simulink model "constraints_comparison_A_4D_v2_Fc_connected"  (R2017b)
settings: Solver=ode4  StartTime=0.0  StopTime=total_time  FixedStep=0.001  RelTol=1e-3  EnableMultiTasking=on
InitFcn:
  | % clear
  | % clc
  | 
  | wavelet_gen
undefined symbols (not defined in the file or in its folder): acm_aero_model, acm_T_N, breakpoints1, Cm0, Cmde, Cmq, comp_feedback, constraint_type, dail, de, dele, dele_trim, drud, FCdelay, firstimpulsewidth3211, firstimpulsewidthdoublet, Fr_mp_1, Fr_mp_2, Fr_rp_1, Fr_rp_2, ini_acm_de_deg, ini_acm_p_deg_per_s, ini_acm_phi_deg, ini_acm_psi_deg, ini_acm_q_deg_per_s, ini_acm_r_deg_per_s, ini_acm_theta_deg, ini_cmp_de_deg, ini_rig_p_deg_per_s, ini_rig_phi_deg, ini_rig_psi_deg, ini_rig_q_deg_per_s, ini_rig_r_deg_per_s, ini_rig_theta_deg, input_type, K1_svo_acm, K1_svo_cmp, K2_svo_acm, K2_svo_cmp, La, Ma, max_defl_sat_acm, max_defl_sat_cmp, max_rate_sat, max_rate_sat_acm, max_rate_sat_cmp, Na, radius, sigbuilder_block, simstop, theta_trim, thrust_trim, windspeed, Xa, Ya, Za
libraries: aerolibconvert2 x119, simulink x36, sharedtransform x19, vrlib x2
(part 3 of 6)

== system constraints_comparison_A_4D_v2_Fc_connected/Control surface input/5) Dutch roll ==
  note: From the lateral_linear_model.m script:
      | The Dutch roll has a damped natural frequency of 12.9511 rad/s (2.0612 Hz)
      | So the period of the mode is: T = 1/2.0612 = 0.4852 seconds
      |
      | From simulation results:
      | T = 0.4825 seconds
      | f = 2.0725 Hz
  note: Trim (wings level):
      | T = 2.037 N
      | dail = 0 deg
      | dele = -1.22537 deg
      | drud = 0 deg
      | phi = 0 deg
      | theta = 1.612 deg
      | psi = 0 deg
      |
      | Trim (phi = -15 deg):
      | T = 2.225 N
      | dail = -30.39 deg
      | dele = -1.382 deg
      | drud = -36.89 deg
      | phi = -15.01 deg
      | theta = 5.134 deg
      | psi = 11.95 deg
      |
      | Trim (phi = -10 deg):
      | T = 2.026 N
      | dail = -18.93 deg
      | dele = -1.148 deg
      | drud = -22.97 deg
      | phi = -10 deg
      | theta = 2.793 deg
      | psi = 7.106 deg
  note: Trim (wings level)
      | NO THRUST:
      | T = 0 N
      | dail = 0 deg
      | dele = -1.2402 deg
      | drud = 0 deg
      | phi = 0 deg
      | theta = 1.632 deg
      | psi = 0 deg
  Angle Conversion : aerolibconvert2/Angle Conversion  IU=deg  OU=rad
  Angle Conversion1 : aerolibconvert2/Angle Conversion  IU=deg  OU=rad
  Angle Conversion2 : aerolibconvert2/Angle Conversion  IU=deg  OU=rad
  Constant : Constant  Value=0
  Constant2 : Constant  Value=0
  From Workspace : FromWorkspace  VariableName=waveletDR  SampleTime=0  OutputAfterFinalValue=Setting to zero
  Gain : Gain  Commented=on  Gain=0.5
  Gain1 : Gain
  Gain8 : Gain  Gain=3
  Mux : Mux  Inputs=3
  Signal Builder : Subsystem  Tag=STV Subsys  Commented=on  LoadFcn=sigbuilder_block('load');  StartFcn=sigbuilder_block('start');  StopFcn=sigbuilder_block('stop');  ClipboardFcn=sigbuilder_block('clipboard');  mask(Sigbuilder block){tuvar=[0:10]}
      mask help: Simulink:masks:SigbuilderBlock_MD
      mask init:
      | if ~strcmp(get_param(bdroot(gcbh),'SimulationStatus'),'stopped') tuvar = sigbuilder_block('maskInit'); end
      settings: CopyFcn=sigbuilder_block('copy');  DeleteFcn=sigbuilder_block('delete');  ModelCloseFcn=sigbuilder_block('modelClose');  PreSaveFcn=sigbuilder_block('preSave');  PauseFcn=sigbuilder_block('pause');  ContinueFcn=sigbuilder_block('continue');  NameChangeFcn=sigbuilder_block('namechange');  OpenFcn=sigbuilder_block('open',[648.75 96.75 712.5 561.75 ]);  CloseFcn=sigbuilder_block('close');
      mask Display: plot(0, 0, 100, 100,[2, 2, 32, 32, 2], [68, 8, 8, 68, 68],[32, 2], [38, 38], [32, 19, 2],[53, 60, 44], [32, 17, 17, 2],[16, 16, 31, 31]);txt = getActiveGroup(gcbh);text(2, 100, txt,'verticalAlignment', 'top');
  Signal Builder1 : Subsystem  Tag=STV Subsys  LoadFcn=sigbuilder_block('load');  StartFcn=sigbuilder_block('start');  StopFcn=sigbuilder_block('stop');  ClipboardFcn=sigbuilder_block('clipboard');  mask(Sigbuilder block){tuvar=[0:10]}
      mask help: Simulink:masks:SigbuilderBlock_MD
      mask init:
      | if ~strcmp(get_param(bdroot(gcbh),'SimulationStatus'),'stopped') tuvar = sigbuilder_block('maskInit'); end
      settings: CopyFcn=sigbuilder_block('copy');  DeleteFcn=sigbuilder_block('delete');  ModelCloseFcn=sigbuilder_block('modelClose');  PreSaveFcn=sigbuilder_block('preSave');  PauseFcn=sigbuilder_block('pause');  ContinueFcn=sigbuilder_block('continue');  NameChangeFcn=sigbuilder_block('namechange');  OpenFcn=sigbuilder_block('open',[715.5 30.75 718.5 675 ]);  CloseFcn=sigbuilder_block('close');
      mask Display: plot(0, 0, 100, 100,[2, 2, 32, 32, 2], [68, 8, 8, 68, 68],[32, 2], [38, 38], [32, 19, 2],[53, 60, 44], [32, 17, 17, 2],[16, 16, 31, 31]);txt = getActiveGroup(gcbh);text(2, 100, txt,'verticalAlignment', 'top');
  Sum : Sum  Inputs=++|
  Sum1 : Sum  Inputs=++|
  Sum2 : Sum  Inputs=++|
  dail_ini : Constant  Value=0
  dele_ini : Constant  Value=-1.2402
  dele_ini1 : Constant  Value=dele_trim
  drud_ini : Constant  Value=0.000000001
  cs_command (rad) : Outport
  wires:
  Angle Conversion2/1 -> Mux/3  "drud"
  Angle Conversion1/1 -> Mux/2  "dele"
  Angle Conversion/1 -> Mux/1  "dail"
  Mux/1 -> cs_command (rad)/1
  Signal Builder1/1(Signal 1) -> Gain1/1
  Signal Builder/1(Signal 1) -> Gain/1
  Constant/1 -> Sum/2
  Gain8/1 -> Sum2/2
  Constant2/1 -> Sum1/2
  dail_ini/1 -> Sum/1
  dele_ini/1 -> ?
  drud_ini/1 -> Sum2/1
  Sum2/1 -> Angle Conversion2/1
  Sum1/1 -> Angle Conversion1/1
  Sum/1 -> Angle Conversion/1
  dele_ini1/1 -> Sum1/1
  From Workspace/1 -> Gain8/1

== system constraints_comparison_A_4D_v2_Fc_connected/Subsystem14/Aerodynamics lookup ==
  Alpha (deg) : Inport
  1-D Lookup Table : Lookup_n-D  NumberOfTableDimensions=1  BreakpointsForDimension1=breakpoints1  Table=de  DiagnosticForOutOfRangeInput=Warning  InternalRulePriority=Speed  RndMeth=Simplest  InputSameDT=on
  1-D Lookup Table1 : Lookup_n-D  NumberOfTableDimensions=1  BreakpointsForDimension1=breakpoints1  Table=Cm0  DiagnosticForOutOfRangeInput=Warning  InternalRulePriority=Speed  RndMeth=Simplest  InputSameDT=on
  1-D Lookup Table2 : Lookup_n-D  NumberOfTableDimensions=1  BreakpointsForDimension1=breakpoints1  Table=Cmde  DiagnosticForOutOfRangeInput=Warning  InternalRulePriority=Speed  RndMeth=Simplest  InputSameDT=on
  1-D Lookup Table3 : Lookup_n-D  NumberOfTableDimensions=1  BreakpointsForDimension1=breakpoints1  Table=Cmq  DiagnosticForOutOfRangeInput=Warning  InternalRulePriority=Speed  RndMeth=Simplest  InputSameDT=on
  Cm0 : Outport
  Cmde : Outport  Port=2
  de_deg : Outport  Port=3
  Cmq : Outport  Port=4
  wires:
  1-D Lookup Table/1 -> de_deg/1  "de_deg"
  1-D Lookup Table1/1 -> Cm0/1  "Cm0"
  Alpha (deg)/1 -> 1-D Lookup Table3/1, 1-D Lookup Table/1, 1-D Lookup Table2/1, 1-D Lookup Table1/1  "Alpha (deg)"
  1-D Lookup Table3/1 -> Cmq/1  "Cmq"
  1-D Lookup Table2/1 -> Cmde/1  "Cmde"

== system constraints_comparison_A_4D_v2_Fc_connected/Subsystem14/Compensator servo model1 ==
  Command : Inport
  Mot : Gain  Gain=K2_svo_cmp
  Saturation : Saturate  UpperLimit=max_rate_sat_cmp  LowerLimit=-max_rate_sat_cmp
  Sum : Sum  Inputs=|+-
  Sum1 : Sum  Inputs=|+-
  Svo : Gain  Gain=K1_svo_cmp
  kinematic : Subsystem
  Response : Outport
  wires:
  Sum/1 -> Svo/1
  Svo/1 -> Saturation/1
  Sum1/1 -> Mot/1
  Saturation/1 -> Sum1/1
  kinematic/1(de) -> Response/1, Sum/2
  Mot/1 -> kinematic/1(rate_dot)
  kinematic/2(de_dot) -> Sum1/2
  Command/1 -> Sum/1

== system constraints_comparison_A_4D_v2_Fc_connected/Subsystem14/Compensator servo model2 ==
  Command : Inport
  Mot : Gain  Gain=K2_svo_cmp
  Saturation : Saturate  UpperLimit=max_rate_sat_cmp  LowerLimit=-max_rate_sat_cmp
  Sum : Sum  Inputs=|+-
  Sum1 : Sum  Inputs=|+-
  Svo : Gain  Gain=K1_svo_cmp
  kinematic : Subsystem
  Response : Outport
  wires:
  Command/1 -> Sum/1
  kinematic/2(de_dot) -> Sum1/2
  Mot/1 -> kinematic/1(rate_dot)
  kinematic/1(de) -> Sum/2, Response/1
  Saturation/1 -> Sum1/1
  Sum1/1 -> Mot/1
  Svo/1 -> Saturation/1
  Sum/1 -> Svo/1

== system constraints_comparison_A_4D_v2_Fc_connected/Subsystem14/Compensator servo model3 ==
  Command : Inport
  Mot : Gain  Gain=K2_svo_cmp
  Saturation : Saturate  UpperLimit=max_rate_sat_cmp  LowerLimit=-max_rate_sat_cmp
  Sum : Sum  Inputs=|+-
  Sum1 : Sum  Inputs=|+-
  Svo : Gain  Gain=K1_svo_cmp
  kinematic : Subsystem
  Response : Outport
  wires:
  Sum/1 -> Svo/1
  Svo/1 -> Saturation/1
  Sum1/1 -> Mot/1
  Saturation/1 -> Sum1/1
  kinematic/1(de) -> Response/1, Sum/2
  Mot/1 -> kinematic/1(rate_dot)
  kinematic/2(de_dot) -> Sum1/2
  Command/1 -> Sum/1

== system constraints_comparison_A_4D_v2_Fc_connected/Subsystem14/Compensator servo model4 ==
  Command : Inport
  Mot : Gain  Gain=K2_svo_cmp
  Saturation : Saturate  UpperLimit=max_rate_sat_cmp  LowerLimit=-max_rate_sat_cmp
  Sum : Sum  Inputs=|+-
  Sum1 : Sum  Inputs=|+-
  Svo : Gain  Gain=K1_svo_cmp
  kinematic : Subsystem
  Response : Outport
  wires:
  Command/1 -> Sum/1
  kinematic/2(de_dot) -> Sum1/2
  Mot/1 -> kinematic/1(rate_dot)
  kinematic/1(de) -> Sum/2, Response/1
  Saturation/1 -> Sum1/1
  Sum1/1 -> Mot/1
  Svo/1 -> Saturation/1
  Sum/1 -> Svo/1

== system constraints_comparison_A_4D_v2_Fc_connected/Subsystem14/Extracting position vector 1 ==
  In1 : Inport
  MATLAB Function : MATLAB Function  TreatAsAtomicUnit=on
  Out1 : Outport
  wires:
  In1/1 -> MATLAB Function/1(u)
  MATLAB Function/1(y) -> Out1/1

== system constraints_comparison_A_4D_v2_Fc_connected/Subsystem14/Extracting position vector 2 ==
  In1 : Inport
  MATLAB Function : MATLAB Function  TreatAsAtomicUnit=on
  Out1 : Outport
  wires:
  In1/1 -> MATLAB Function/1(u)
  MATLAB Function/1(y) -> Out1/1

== system constraints_comparison_A_4D_v2_Fc_connected/Subsystem14/Extracting position vector 2  ==
  In1 : Inport
  MATLAB Function : MATLAB Function  TreatAsAtomicUnit=on
  Out1 : Outport
  wires:
  MATLAB Function/1(y) -> Out1/1
  In1/1 -> MATLAB Function/1(u)

== system constraints_comparison_A_4D_v2_Fc_connected/Subsystem14/Extracting position vector 3 ==
  In1 : Inport
  MATLAB Function : MATLAB Function  TreatAsAtomicUnit=on
  Out1 : Outport
  wires:
  In1/1 -> MATLAB Function/1(u)
  MATLAB Function/1(y) -> Out1/1

== system constraints_comparison_A_4D_v2_Fc_connected/Subsystem14/Extracting position vector 4 ==
  In1 : Inport
  MATLAB Function : MATLAB Function  TreatAsAtomicUnit=on
  Out1 : Outport
  wires:
  MATLAB Function/1(y) -> Out1/1
  In1/1 -> MATLAB Function/1(u)

== system constraints_comparison_A_4D_v2_Fc_connected/Subsystem14/Extracting position vector 5 ==
  In1 : Inport
  MATLAB Function : MATLAB Function  TreatAsAtomicUnit=on
  Out1 : Outport
  wires:
  MATLAB Function/1(y) -> Out1/1
  In1/1 -> MATLAB Function/1(u)

== system constraints_comparison_A_4D_v2_Fc_connected/Subsystem14/Hawk servo model ==
  note: Above saturation
      | represents voltage
      | saturation
  Command : Inport
  Mot : Gain  Gain=K2_svo_acm
  Saturation : Saturate  UpperLimit=max_rate_sat_acm  LowerLimit=-max_rate_sat_acm
  Sum : Sum  Inputs=|+-
  Sum1 : Sum  Inputs=|+-
  Svo : Gain  Gain=K1_svo_acm
  kinematic : Subsystem
  Response : Outport
  wires:
  Sum/1 -> Svo/1
  Svo/1 -> Saturation/1
  Sum1/1 -> Mot/1
  Saturation/1 -> Sum1/1
  kinematic/1(de) -> Response/1, Sum/2
  Mot/1 -> kinematic/1(rate_dot)
  kinematic/2(de_dot) -> Sum1/2
  Command/1 -> Sum/1

== system constraints_comparison_A_4D_v2_Fc_connected/Subsystem14/Signal Builder ==
  Demux : Demux  Tag=STV Demux  Outputs=1
  FromWs : FromWorkspace  Tag=STV FromWs  VariableName=tuvar  SampleTime=0
      SigBuilderData=|
      | common.afterFinalStr = 'Extrapolate'
      | common.sampleTime = 0
      | dataSet.timeRange = [0 10]
      | dataSet.name = 'Group 1'
      | sbobj.Groups.Name = 'Group 1'
      | sbobj.Groups.Signals.Name = 'Signal 1'
      | sbobj.Groups.Signals.XData = [0 1 1 1.1 1.1 1.2 1.2 10]
      | sbobj.Groups.Signals.YData = [0 0 1 1 -1 -1 0 0]
  Signal 1 : Outport  Tag=STV Outport
  wires:
  Demux/1 -> Signal 1/1
  FromWs/1 -> Demux/1

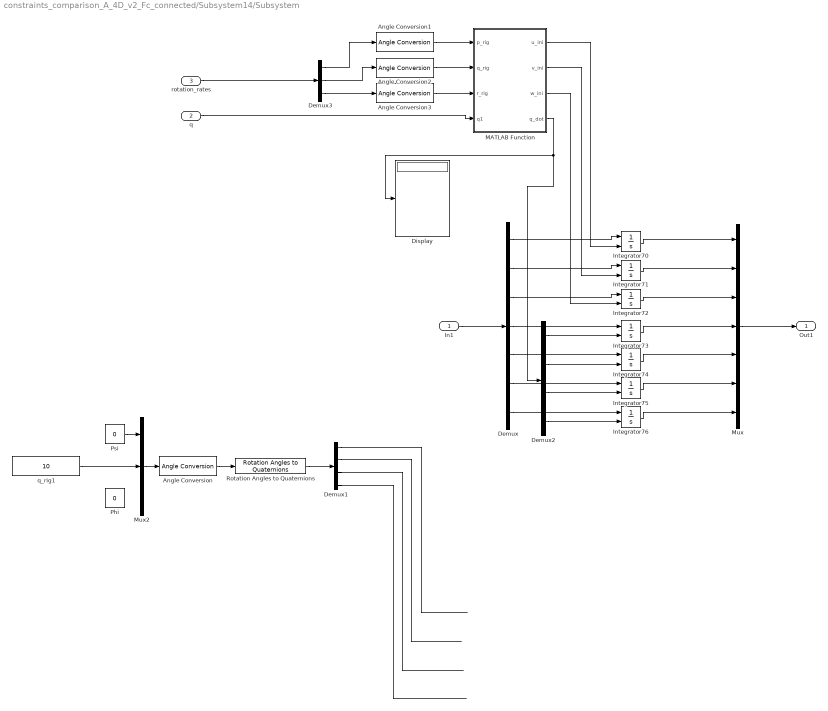
== system constraints_comparison_A_4D_v2_Fc_connected/Subsystem14/Subsystem ==
  In1 : Inport
  q : Inport  Port=2
  rotation_rates : Inport  Port=3
  Angle Conversion{,1..3} (4 alike) : aerolibconvert2/Angle Conversion  IU=deg  OU=rad
  Demux : Demux  Outputs=7
  Demux1 : Demux
  Demux2 : Demux
  Demux3 : Demux  Outputs=3
  Display : Display
  Integrator{70..76} (7 alike) : Integrator  InitialConditionSource=external
  MATLAB Function : MATLAB Function
  Mux : Mux  Inputs=7
  Mux2 : Mux  Inputs=3
  Phi : Constant  Value=0
  Psi : Constant  Value=0
  Rotation Angles to Quaternions : sharedtransform/Rotation Angles to Quaternions  rotationOrder=ZYX
      settings: SourceProductName=Aerospace Blockset  SourceProductBaseCode=AE
  q_rig1 : Constant  Value=10
  Out1 : Outport
  wires:
  Integrator70/1 -> Mux/1
  Integrator71/1 -> Mux/2
  Integrator72/1 -> Mux/3
  Integrator73/1 -> Mux/4
  Integrator74/1 -> Mux/5
  Integrator75/1 -> Mux/6
  Integrator76/1 -> Mux/7
  Demux/1 -> Integrator70/1
  Demux/7 -> Integrator76/1
  Demux/2 -> Integrator71/1
  Demux/3 -> Integrator72/1
  Demux/4 -> Integrator73/1
  Demux/5 -> Integrator74/1
  Demux/6 -> Integrator75/1
  In1/1 -> Demux/1
  Mux/1 -> Out1/1
  MATLAB Function/1(u_ini) -> Integrator70/2
  MATLAB Function/2(v_ini) -> Integrator71/2
  MATLAB Function/3(w_ini) -> Integrator72/2
  rotation_rates/1 -> Demux3/1
  Psi/1 -> Mux2/1
  Mux2/1 -> Angle Conversion/1
  Rotation Angles to Quaternions/1 -> Demux1/1
  Demux1/4 -> ?
  Demux1/1 -> ?
  Demux1/2 -> ?
  Demux1/3 -> ?
  Angle Conversion/1 -> Rotation Angles to Quaternions/1
  Angle Conversion2/1 -> MATLAB Function/2(q_rig)
  q_rig1/1 -> Mux2/2
  q/1 -> MATLAB Function/4(q1)
  Demux2/1 -> Integrator73/2
  Demux2/2 -> Integrator74/2
  Demux2/3 -> Integrator75/2
  Demux2/4 -> Integrator76/2
  MATLAB Function/4(q_dot) -> Demux2/1, Display/1
  Demux3/2 -> Angle Conversion2/1
  Demux3/1 -> Angle Conversion1/1
  Angle Conversion1/1 -> MATLAB Function/1(p_rig)
  Demux3/3 -> Angle Conversion3/1
  Angle Conversion3/1 -> MATLAB Function/3(r_rig)

== system constraints_comparison_A_4D_v2_Fc_connected/Subsystem14/Subsystem1 ==
  In1 : Inport
  rig attitude : Inport  Port=2
  Angle Conversion : aerolibconvert2/Angle Conversion  IU=deg  OU=rad
  Demux : Demux  Outputs=7
  Demux1 : Demux
  Display : Display
  Display1 : Display
  Display2 : Display
  Integrator70 : Integrator  InitialConditionSource=external  InitialCondition=-0.38
  Integrator{71..72,74..76} (5 alike) : Integrator  InitialConditionSource=external
  Integrator73 : Integrator  InitialConditionSource=external  InitialCondition=1
  MATLAB Function : MATLAB Function
  Mux : Mux  Inputs=7
  Quaternions to Rotation Angles : sharedtransform/Quaternions to Rotation Angles  rotationOrder=ZYX
      settings: SourceProductBaseCode=AE
  Rotation Angles to Quaternions : sharedtransform/Rotation Angles to Quaternions  rotationOrder=ZYX
      settings: SourceProductName=Aerospace Blockset  SourceProductBaseCode=AE
  Out1 : Outport
  wires:
  Mux/1 -> Out1/1
  In1/1 -> Demux/1
  Demux/6 -> Integrator75/1
  Demux/5 -> Integrator74/1
  Demux/4 -> Integrator73/1
  Demux/3 -> Integrator72/1
  Demux/2 -> Integrator71/1
  Demux/7 -> Integrator76/1
  Demux/1 -> Integrator70/1
  Integrator76/1 -> Mux/7
  Integrator75/1 -> Mux/6
  Integrator74/1 -> Mux/5
  Integrator73/1 -> Mux/4
  Integrator72/1 -> Mux/3
  Integrator71/1 -> Mux/2
  Integrator70/1 -> Mux/1
  MATLAB Function/1(x_ini) -> Integrator70/2
  MATLAB Function/2(y_ini) -> Integrator71/2
  MATLAB Function/3(z_ini) -> Integrator72/2
  rig attitude/1 -> Angle Conversion/1
  Demux1/4 -> Integrator76/2
  Demux1/1 -> Integrator73/2
  Demux1/2 -> Integrator74/2
  Demux1/3 -> Integrator75/2
  Angle Conversion/1 -> Display1/1, Rotation Angles to Quaternions/1
  Rotation Angles to Quaternions/1 -> Quaternions to Rotation Angles/1, Display/1, MATLAB Function/1(q), Demux1/1
  Quaternions to Rotation Angles/1 -> Display2/1

== system constraints_comparison_A_4D_v2_Fc_connected/Subsystem14/Subsystem10 ==
  In1 : Inport
  q : Inport  Port=2
  rotation_rates : Inport  Port=3
  Angle Conversion1 : aerolibconvert2/Angle Conversion  IU=deg  OU=rad
  Angle Conversion2 : aerolibconvert2/Angle Conversion  IU=deg  OU=rad
  Angle Conversion3 : aerolibconvert2/Angle Conversion  IU=deg  OU=rad
  Demux : Demux  Outputs=7
  Demux1 : Demux
  Demux3 : Demux  Outputs=3
  Display : Display
  Integrator{70..76} (7 alike) : Integrator  InitialConditionSource=external
  MATLAB Function : MATLAB Function
  Mux : Mux  Inputs=7
  Out1 : Outport
  wires:
  Integrator70/1 -> Mux/1
  Integrator71/1 -> Mux/2
  Integrator72/1 -> Mux/3
  Integrator73/1 -> Mux/4
  Integrator74/1 -> Mux/5
  Integrator75/1 -> Mux/6
  Integrator76/1 -> Mux/7
  Demux/1 -> Integrator70/1
  Demux/7 -> Integrator76/1
  Demux/2 -> Integrator71/1
  Demux/3 -> Integrator72/1
  Demux/4 -> Integrator73/1
  Demux/5 -> Integrator74/1
  Demux/6 -> Integrator75/1
  In1/1 -> Demux/1
  Mux/1 -> Out1/1
  MATLAB Function/1(u_ini) -> Integrator70/2
  MATLAB Function/2(v_ini) -> Integrator71/2
  MATLAB Function/3(w_ini) -> Integrator72/2
  rotation_rates/1 -> Demux3/1
  Angle Conversion1/1 -> MATLAB Function/1(p_rig)
  Angle Conversion2/1 -> MATLAB Function/2(q_rig)
  q/1 -> MATLAB Function/4(q1)
  MATLAB Function/4(q_dot) -> Demux1/1, Display/1
  Demux1/4 -> Integrator76/2
  Demux1/3 -> Integrator75/2
  Demux1/2 -> Integrator74/2
  Demux1/1 -> Integrator73/2
  Angle Conversion3/1 -> MATLAB Function/3(r_rig)
  Demux3/3 -> Angle Conversion3/1
  Demux3/2 -> Angle Conversion2/1
  Demux3/1 -> Angle Conversion1/1

== system constraints_comparison_A_4D_v2_Fc_connected/Subsystem14/Subsystem11 ==
  In1 : Inport
  rig attitude : Inport  Port=2
  Angle Conversion : aerolibconvert2/Angle Conversion  IU=deg  OU=rad
  Demux : Demux  Outputs=7
  Demux1 : Demux
  Display : Display
  Integrator70 : Integrator  InitialConditionSource=external  InitialCondition=0.8
  Integrator{71,74..76} (4 alike) : Integrator  InitialConditionSource=external
  Integrator72 : Integrator  InitialConditionSource=external  InitialCondition=0.3183
  Integrator73 : Integrator  InitialConditionSource=external  InitialCondition=1
  MATLAB Function : MATLAB Function
  Mux : Mux  Inputs=7
  Rotation Angles to Quaternions : sharedtransform/Rotation Angles to Quaternions  rotationOrder=ZYX
      settings: SourceProductName=Aerospace Blockset  SourceProductBaseCode=AE
  Terminator : Terminator
  Theta : Constant  Value=0
  Out1 : Outport
  wires:
  Mux/1 -> Out1/1
  In1/1 -> Demux/1
  Demux/6 -> Integrator75/1
  Demux/5 -> Integrator74/1
  Demux/4 -> Integrator73/1
  Demux/3 -> Integrator72/1
  Demux/2 -> Integrator71/1
  Demux/7 -> Integrator76/1
  Demux/1 -> Integrator70/1
  Integrator76/1 -> Mux/7
  Integrator75/1 -> Mux/6
  Integrator74/1 -> Mux/5
  Integrator73/1 -> Mux/4
  Integrator72/1 -> Mux/3
  Integrator71/1 -> Mux/2
  Integrator70/1 -> Mux/1
  Theta/1 -> Terminator/1
  Rotation Angles to Quaternions/1 -> Demux1/1, MATLAB Function/1(q), Display/1
  Demux1/4 -> Integrator76/2
  Demux1/1 -> Integrator73/2
  Demux1/2 -> Integrator74/2
  Demux1/3 -> Integrator75/2
  Angle Conversion/1 -> Rotation Angles to Quaternions/1
  MATLAB Function/1(x_ini) -> Integrator70/2
  MATLAB Function/2(y_ini) -> Integrator71/2
  MATLAB Function/3(z_ini) -> Integrator72/2
  rig attitude/1 -> Angle Conversion/1

== system constraints_comparison_A_4D_v2_Fc_connected/Subsystem14/Subsystem12 ==
  In1 : Inport
  q : Inport  Port=2
  rotation_rates : Inport  Port=3
  Angle Conversion1 : aerolibconvert2/Angle Conversion  IU=deg  OU=rad
  Angle Conversion2 : aerolibconvert2/Angle Conversion  IU=deg  OU=rad
  Angle Conversion3 : aerolibconvert2/Angle Conversion  IU=deg  OU=rad
  Demux : Demux  Outputs=7
  Demux1 : Demux
  Demux3 : Demux  Outputs=3
  Display : Display
  Integrator{70..76} (7 alike) : Integrator  InitialConditionSource=external
  MATLAB Function : MATLAB Function
  Mux : Mux  Inputs=7
  Out1 : Outport
  wires:
  Demux1/1 -> Integrator73/2
  Demux1/2 -> Integrator74/2
  Demux1/3 -> Integrator75/2
  Demux1/4 -> Integrator76/2
  MATLAB Function/4(q_dot) -> Display/1, Demux1/1
  q/1 -> MATLAB Function/4(q1)
  Angle Conversion2/1 -> MATLAB Function/2(q_rig)
  Angle Conversion1/1 -> MATLAB Function/1(p_rig)
  rotation_rates/1 -> Demux3/1
  MATLAB Function/3(w_ini) -> Integrator72/2
  MATLAB Function/2(v_ini) -> Integrator71/2
  MATLAB Function/1(u_ini) -> Integrator70/2
  Mux/1 -> Out1/1
  In1/1 -> Demux/1
  Demux/6 -> Integrator75/1
  Demux/5 -> Integrator74/1
  Demux/4 -> Integrator73/1
  Demux/3 -> Integrator72/1
  Demux/2 -> Integrator71/1
  Demux/7 -> Integrator76/1
  Demux/1 -> Integrator70/1
  Integrator76/1 -> Mux/7
  Integrator75/1 -> Mux/6
  Integrator74/1 -> Mux/5
  Integrator73/1 -> Mux/4
  Integrator72/1 -> Mux/3
  Integrator71/1 -> Mux/2
  Integrator70/1 -> Mux/1
  Angle Conversion3/1 -> MATLAB Function/3(r_rig)
  Demux3/3 -> Angle Conversion3/1
  Demux3/2 -> Angle Conversion2/1
  Demux3/1 -> Angle Conversion1/1

== system constraints_comparison_A_4D_v2_Fc_connected/Subsystem14/Subsystem13 ==
  In1 : Inport
  rig attitude : Inport  Port=2
  Angle Conversion : aerolibconvert2/Angle Conversion  IU=deg  OU=rad
  Demux : Demux  Outputs=7
  Demux1 : Demux
  Display : Display
  Integrator70 : Integrator  InitialConditionSource=external  InitialCondition=0.8
  Integrator{71,74..76} (4 alike) : Integrator  InitialConditionSource=external
  Integrator72 : Integrator  InitialConditionSource=external  InitialCondition=0.1433
  Integrator73 : Integrator  InitialConditionSource=external  InitialCondition=1
  MATLAB Function : MATLAB Function
  Mux : Mux  Inputs=7
  Rotation Angles to Quaternions : sharedtransform/Rotation Angles to Quaternions  rotationOrder=ZYX
      settings: SourceProductName=Aerospace Blockset  SourceProductBaseCode=AE
  Out1 : Outport
  wires:
  Angle Conversion/1 -> Rotation Angles to Quaternions/1
  Demux1/3 -> Integrator75/2
  Demux1/2 -> Integrator74/2
  Demux1/1 -> Integrator73/2
  Demux1/4 -> Integrator76/2
  Integrator70/1 -> Mux/1
  Integrator71/1 -> Mux/2
  Integrator72/1 -> Mux/3
  Integrator73/1 -> Mux/4
  Integrator74/1 -> Mux/5
  Integrator75/1 -> Mux/6
  Integrator76/1 -> Mux/7
  Demux/1 -> Integrator70/1
  Demux/7 -> Integrator76/1
  Demux/2 -> Integrator71/1
  Demux/3 -> Integrator72/1
  Demux/4 -> Integrator73/1
  Demux/5 -> Integrator74/1
  Demux/6 -> Integrator75/1
  In1/1 -> Demux/1
  Mux/1 -> Out1/1
  MATLAB Function/3(z_ini) -> Integrator72/2
  Rotation Angles to Quaternions/1 -> MATLAB Function/1(q), Display/1, Demux1/1
  MATLAB Function/1(x_ini) -> Integrator70/2
  MATLAB Function/2(y_ini) -> Integrator71/2
  rig attitude/1 -> Angle Conversion/1

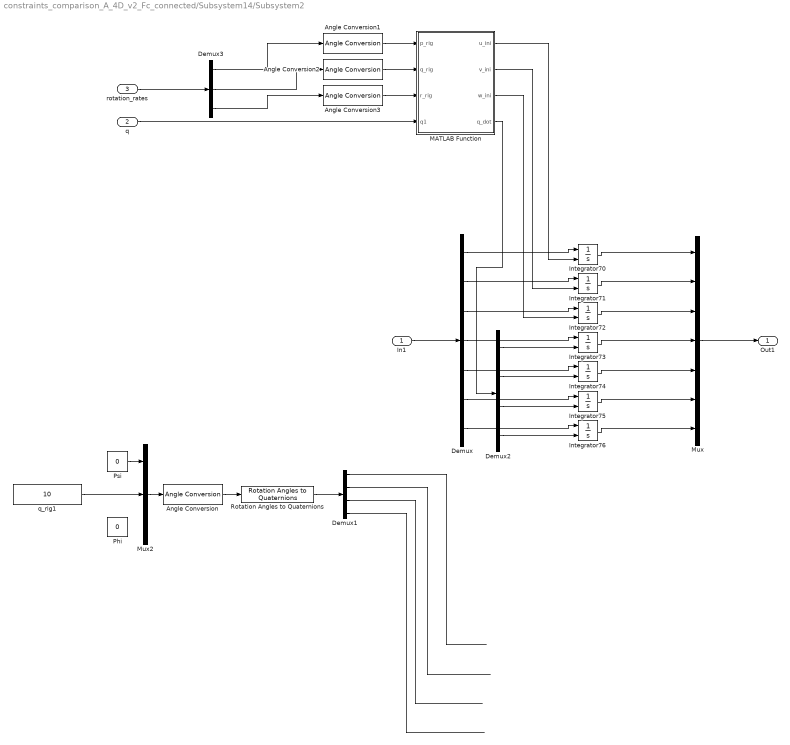
== system constraints_comparison_A_4D_v2_Fc_connected/Subsystem14/Subsystem2 ==
  In1 : Inport
  q : Inport  Port=2
  rotation_rates : Inport  Port=3
  Angle Conversion{,1..3} (4 alike) : aerolibconvert2/Angle Conversion  IU=deg  OU=rad
  Demux : Demux  Outputs=7
  Demux1 : Demux
  Demux2 : Demux
  Demux3 : Demux  Outputs=3
  Integrator{70..76} (7 alike) : Integrator  InitialConditionSource=external
  MATLAB Function : MATLAB Function
  Mux : Mux  Inputs=7
  Mux2 : Mux  Inputs=3
  Phi : Constant  Value=0
  Psi : Constant  Value=0
  Rotation Angles to Quaternions : sharedtransform/Rotation Angles to Quaternions  rotationOrder=ZYX
      settings: SourceProductName=Aerospace Blockset  SourceProductBaseCode=AE
  q_rig1 : Constant  Value=10
  Out1 : Outport
  wires:
  Mux/1 -> Out1/1
  In1/1 -> Demux/1
  Demux/6 -> Integrator75/1
  Demux/5 -> Integrator74/1
  Demux/4 -> Integrator73/1
  Demux/3 -> Integrator72/1
  Demux/2 -> Integrator71/1
  Demux/7 -> Integrator76/1
  Demux/1 -> Integrator70/1
  Integrator76/1 -> Mux/7
  Integrator75/1 -> Mux/6
  Integrator74/1 -> Mux/5
  Integrator73/1 -> Mux/4
  Integrator72/1 -> Mux/3
  Integrator71/1 -> Mux/2
  Integrator70/1 -> Mux/1
  MATLAB Function/1(u_ini) -> Integrator70/2
  MATLAB Function/2(v_ini) -> Integrator71/2
  MATLAB Function/3(w_ini) -> Integrator72/2
  Angle Conversion1/1 -> MATLAB Function/1(p_rig)
  Angle Conversion2/1 -> MATLAB Function/2(q_rig)
  rotation_rates/1 -> Demux3/1
  Psi/1 -> Mux2/1
  Mux2/1 -> Angle Conversion/1
  Rotation Angles to Quaternions/1 -> Demux1/1
  Demux1/4 -> ?
  Demux1/1 -> ?
  Demux1/2 -> ?
  Demux1/3 -> ?
  Angle Conversion/1 -> Rotation Angles to Quaternions/1
  q_rig1/1 -> Mux2/2
  q/1 -> MATLAB Function/4(q1)
  Demux2/1 -> Integrator73/2
  Demux2/2 -> Integrator74/2
  Demux2/3 -> Integrator75/2
  Demux2/4 -> Integrator76/2
  MATLAB Function/4(q_dot) -> Demux2/1
  Demux3/1 -> Angle Conversion1/1
  Demux3/2 -> Angle Conversion2/1
  Angle Conversion3/1 -> MATLAB Function/3(r_rig)
  Demux3/3 -> Angle Conversion3/1

== system constraints_comparison_A_4D_v2_Fc_connected/Subsystem14/Subsystem3 ==
  note: Initial angle of attack -->
  In1 : Inport
  rig attitude : Inport  Port=2
  Angle Conversion : aerolibconvert2/Angle Conversion  IU=deg  OU=rad
  Demux : Demux  Outputs=7
  Demux1 : Demux
  Integrator70 : Integrator  InitialConditionSource=external  InitialCondition=0.2615
  Integrator{71,74..76} (4 alike) : Integrator  InitialConditionSource=external
  Integrator72 : Integrator  InitialConditionSource=external  InitialCondition=0.109
  Integrator73 : Integrator  InitialConditionSource=external  InitialCondition=1
  MATLAB Function : MATLAB Function
  Mux : Mux  Inputs=7
  Rotation Angles to Quaternions : sharedtransform/Rotation Angles to Quaternions  rotationOrder=ZYX
      settings: SourceProductName=Aerospace Blockset  SourceProductBaseCode=AE
  Theta : Constant  Value=0
  Out1 : Outport
  wires:
  Integrator70/1 -> Mux/1
  Integrator71/1 -> Mux/2
  Integrator72/1 -> Mux/3
  Integrator73/1 -> Mux/4
  Integrator74/1 -> Mux/5
  Integrator75/1 -> Mux/6
  Integrator76/1 -> Mux/7
  Demux/1 -> Integrator70/1
  Demux/7 -> Integrator76/1
  Demux/2 -> Integrator71/1
  Demux/3 -> Integrator72/1
  Demux/4 -> Integrator73/1
  Demux/5 -> Integrator74/1
  Demux/6 -> Integrator75/1
  In1/1 -> Demux/1
  Mux/1 -> Out1/1
  MATLAB Function/1(x_ini) -> Integrator70/2
  MATLAB Function/2(y_ini) -> Integrator71/2
  MATLAB Function/3(z_ini) -> Integrator72/2
  Demux1/4 -> Integrator76/2
  Demux1/1 -> Integrator73/2
  Demux1/2 -> Integrator74/2
  Demux1/3 -> Integrator75/2
  Angle Conversion/1 -> Rotation Angles to Quaternions/1
  Rotation Angles to Quaternions/1 -> MATLAB Function/1(q), Demux1/1
  rig attitude/1 -> Angle Conversion/1

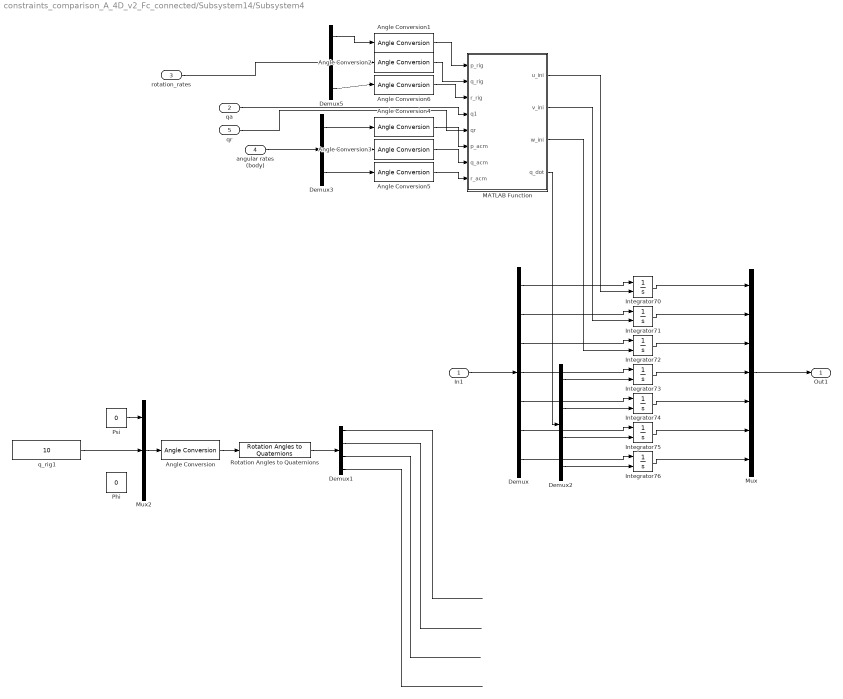
== system constraints_comparison_A_4D_v2_Fc_connected/Subsystem14/Subsystem4 ==
  In1 : Inport
  qa : Inport  Port=2
  rotation_rates : Inport  Port=3
  angular rates (body) : Inport  Port=4
  qr : Inport  Port=5
  Angle Conversion{,1..6} (7 alike) : aerolibconvert2/Angle Conversion  IU=deg  OU=rad
  Demux : Demux  Outputs=7
  Demux1 : Demux
  Demux2 : Demux
  Demux3 : Demux  Outputs=3
  Demux5 : Demux  Outputs=3
  Integrator{70..76} (7 alike) : Integrator  InitialConditionSource=external
  MATLAB Function : MATLAB Function
  Mux : Mux  Inputs=7
  Mux2 : Mux  Inputs=3
  Phi : Constant  Value=0
  Psi : Constant  Value=0
  Rotation Angles to Quaternions : sharedtransform/Rotation Angles to Quaternions  rotationOrder=ZYX
      settings: SourceProductName=Aerospace Blockset  SourceProductBaseCode=AE
  q_rig1 : Constant  Value=10
  Out1 : Outport
  wires:
  Integrator70/1 -> Mux/1
  Integrator71/1 -> Mux/2
  Integrator72/1 -> Mux/3
  Integrator73/1 -> Mux/4
  Integrator74/1 -> Mux/5
  Integrator75/1 -> Mux/6
  Integrator76/1 -> Mux/7
  Demux/1 -> Integrator70/1
  Demux/7 -> Integrator76/1
  Demux/2 -> Integrator71/1
  Demux/3 -> Integrator72/1
  Demux/4 -> Integrator73/1
  Demux/5 -> Integrator74/1
  Demux/6 -> Integrator75/1
  In1/1 -> Demux/1
  Mux/1 -> Out1/1
  MATLAB Function/1(u_ini) -> Integrator70/2
  MATLAB Function/2(v_ini) -> Integrator71/2
  MATLAB Function/3(w_ini) -> Integrator72/2
  Angle Conversion1/1 -> MATLAB Function/1(p_rig)
  Angle Conversion2/1 -> MATLAB Function/2(q_rig)
  rotation_rates/1 -> Demux5/1
  Psi/1 -> Mux2/1
  Mux2/1 -> Angle Conversion/1
  Rotation Angles to Quaternions/1 -> Demux1/1
  Demux1/4 -> ?
  Demux1/1 -> ?
  Demux1/2 -> ?
  Demux1/3 -> ?
  Angle Conversion/1 -> Rotation Angles to Quaternions/1
  q_rig1/1 -> Mux2/2
  qa/1 -> MATLAB Function/4(q1)
  Demux2/1 -> Integrator73/2
  Demux2/2 -> Integrator74/2
  Demux2/3 -> Integrator75/2
  Demux2/4 -> Integrator76/2
  MATLAB Function/4(q_dot) -> Demux2/1
  Angle Conversion3/1 -> MATLAB Function/7(q_acm)
  angular rates (body)/1 -> Demux3/1
  Angle Conversion4/1 -> MATLAB Function/6(p_acm)
  Angle Conversion5/1 -> MATLAB Function/8(r_acm)
  Demux3/3 -> Angle Conversion5/1
  Demux3/1 -> Angle Conversion4/1
  Demux3/2 -> Angle Conversion3/1
  Angle Conversion6/1 -> MATLAB Function/3(r_rig)
  Demux5/1 -> Angle Conversion1/1
  Demux5/2 -> Angle Conversion2/1
  Demux5/3 -> Angle Conversion6/1
  qr/1 -> MATLAB Function/5(qr)

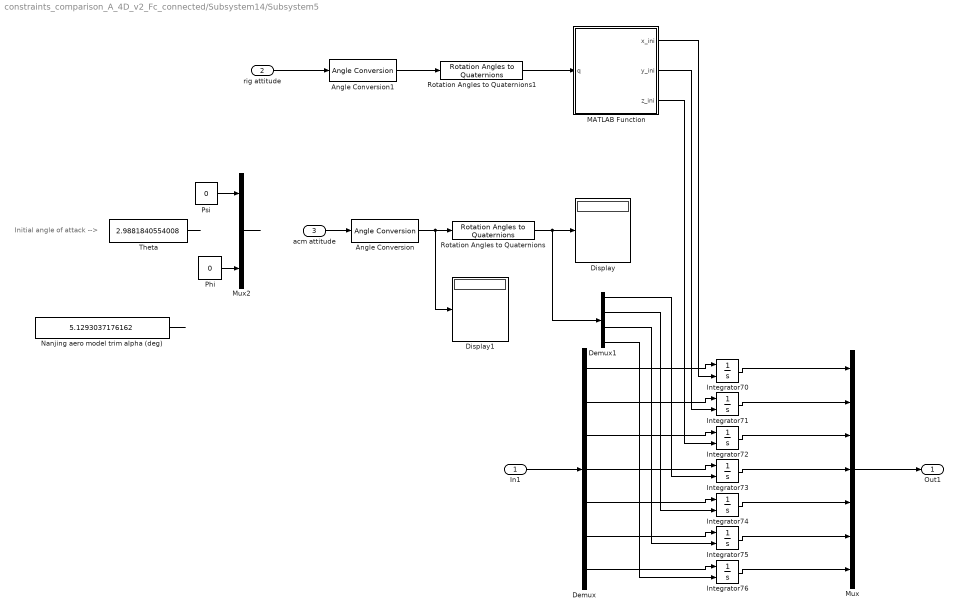
== system constraints_comparison_A_4D_v2_Fc_connected/Subsystem14/Subsystem5 ==
  note: Initial angle of attack -->
  In1 : Inport
  rig attitude : Inport  Port=2
  acm attitude : Inport  Port=3
  Angle Conversion : aerolibconvert2/Angle Conversion  IU=deg  OU=rad
  Angle Conversion1 : aerolibconvert2/Angle Conversion  IU=deg  OU=rad
  Demux : Demux  Outputs=7
  Demux1 : Demux
  Display : Display
  Display1 : Display
  Integrator70 : Integrator  InitialConditionSource=external  InitialCondition=0.8
  Integrator{71..72,74..76} (5 alike) : Integrator  InitialConditionSource=external
  Integrator73 : Integrator  InitialConditionSource=external  InitialCondition=1
  MATLAB Function : MATLAB Function
  Mux : Mux  Inputs=7
  Mux2 : Mux  Inputs=3
  Nanjing aero model trim alpha (deg) : Constant  Value=5.1293037176162
  Phi : Constant  Value=0
  Psi : Constant  Value=0
  Rotation Angles to Quaternions : sharedtransform/Rotation Angles to Quaternions  rotationOrder=ZYX
      settings: SourceProductName=Aerospace Blockset  SourceProductBaseCode=AE
  Rotation Angles to Quaternions1 : sharedtransform/Rotation Angles to Quaternions  rotationOrder=ZYX
      settings: SourceProductName=Aerospace Blockset  SourceProductBaseCode=AE
  Theta : Constant  Value=2.9881840554008
  Out1 : Outport
  wires:
  Mux/1 -> Out1/1
  In1/1 -> Demux/1
  Demux/6 -> Integrator75/1
  Demux/5 -> Integrator74/1
  Demux/4 -> Integrator73/1
  Demux/3 -> Integrator72/1
  Demux/2 -> Integrator71/1
  Demux/7 -> Integrator76/1
  Demux/1 -> Integrator70/1
  Integrator76/1 -> Mux/7
  Integrator75/1 -> Mux/6
  Integrator74/1 -> Mux/5
  Integrator73/1 -> Mux/4
  Integrator72/1 -> Mux/3
  Integrator71/1 -> Mux/2
  Integrator70/1 -> Mux/1
  Phi/1 -> Mux2/3
  Psi/1 -> Mux2/1
  Mux2/1 -> ?
  Rotation Angles to Quaternions/1 -> Demux1/1, Display/1
  Demux1/4 -> Integrator76/2
  Demux1/1 -> Integrator73/2
  Demux1/2 -> Integrator74/2
  Demux1/3 -> Integrator75/2
  Angle Conversion/1 -> Display1/1, Rotation Angles to Quaternions/1
  Nanjing aero model trim alpha (deg)/1 -> ?
  MATLAB Function/1(x_ini) -> Integrator70/2
  MATLAB Function/2(y_ini) -> Integrator71/2
  MATLAB Function/3(z_ini) -> Integrator72/2
  Theta/1 -> ?
  Angle Conversion1/1 -> Rotation Angles to Quaternions1/1
  rig attitude/1 -> Angle Conversion1/1
  acm attitude/1 -> Angle Conversion/1
  Rotation Angles to Quaternions1/1 -> MATLAB Function/1(q)

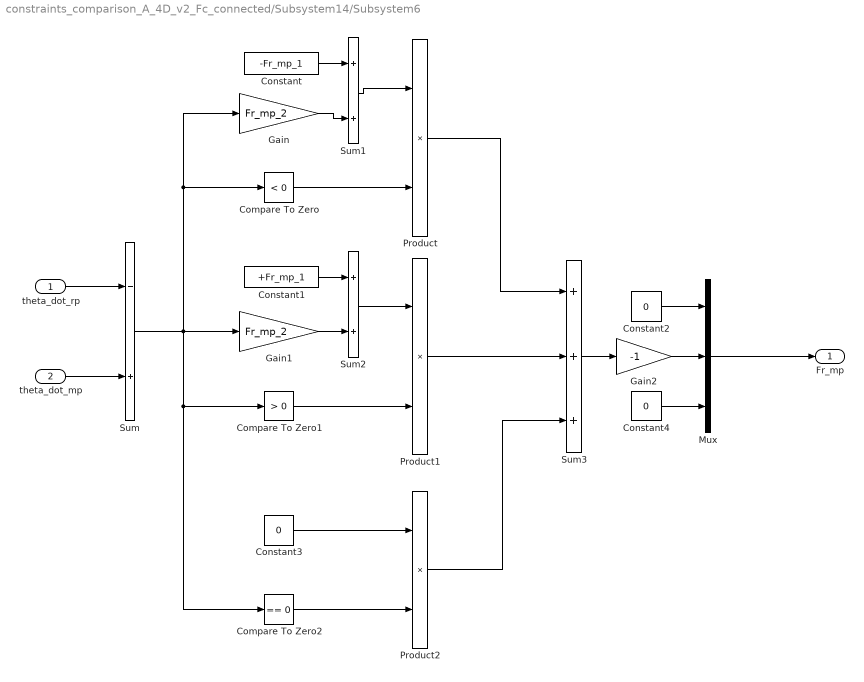
== system constraints_comparison_A_4D_v2_Fc_connected/Subsystem14/Subsystem6 ==
  theta_dot_rp : Inport
  theta_dot_mp : Inport  Port=2
  Compare To Zero : simulink/Logic and Bit Operations/Compare To Zero  relop=<  OutDataTypeStr=boolean
  Compare To Zero1 : simulink/Logic and Bit Operations/Compare To Zero  relop=>  OutDataTypeStr=boolean
  Compare To Zero2 : simulink/Logic and Bit Operations/Compare To Zero  relop===  OutDataTypeStr=boolean
  Constant : Constant  Value=-Fr_mp_1
  Constant1 : Constant  Value=+Fr_mp_1
  Constant2 : Constant  Value=0
  Constant3 : Constant  Value=0
  Constant4 : Constant  Value=0
  Gain : Gain  Gain=Fr_mp_2
  Gain1 : Gain  Gain=Fr_mp_2
  Gain2 : Gain  Gain=-1
  Mux : Mux  Inputs=3
  Product : Product
  Product1 : Product
  Product2 : Product
  Sum : Sum  Inputs=-+
  Sum1 : Sum
  Sum2 : Sum
  Sum3 : Sum  Inputs=+++
  Fr_mp : Outport
  wires:
  theta_dot_rp/1 -> Sum/1
  theta_dot_mp/1 -> Sum/2
  Compare To Zero/1 -> Product/2
  Compare To Zero1/1 -> Product1/2
  Constant/1 -> Sum1/1
  Gain/1 -> Sum1/2
  Sum/1 -> Gain/1, Compare To Zero/1, Compare To Zero2/1, Compare To Zero1/1, Gain1/1
  Sum1/1 -> Product/1
  Constant1/1 -> Sum2/1
  Gain1/1 -> Sum2/2
  Sum2/1 -> Product1/1
  Compare To Zero2/1 -> Product2/2
  Constant4/1 -> Mux/3
  Constant2/1 -> Mux/1
  Mux/1 -> Fr_mp/1
  Constant3/1 -> Product2/1
  Product/1 -> Sum3/1
  Product1/1 -> Sum3/2
  Product2/1 -> Sum3/3
  Sum3/1 -> Gain2/1
  Gain2/1 -> Mux/2

== system constraints_comparison_A_4D_v2_Fc_connected/Subsystem14/Subsystem7 ==
  theta_dot_rp : Inport
  Compare To Zero : simulink/Logic and Bit Operations/Compare To Zero  relop=<  OutDataTypeStr=boolean
  Compare To Zero1 : simulink/Logic and Bit Operations/Compare To Zero  relop=>  OutDataTypeStr=boolean
  Compare To Zero2 : simulink/Logic and Bit Operations/Compare To Zero  relop===  OutDataTypeStr=boolean
  Constant : Constant  Value=-Fr_rp_1
  Constant1 : Constant  Value=+Fr_rp_1
  Constant2 : Constant  Value=0
  Constant3 : Constant  Value=0
  Constant4 : Constant  Value=0
  Gain : Gain  Gain=Fr_rp_2
  Gain1 : Gain  Gain=Fr_rp_2
  Gain2 : Gain  Gain=-1
  Mux : Mux  Inputs=3
  Product : Product
  Product1 : Product
  Product2 : Product
  Sum1 : Sum
  Sum2 : Sum
  Sum3 : Sum  Inputs=+++
  Fr_mp : Outport
  wires:
  Gain2/1 -> Mux/2
  Sum3/1 -> Gain2/1
  Product2/1 -> Sum3/3
  Product1/1 -> Sum3/2
  Product/1 -> Sum3/1
  Constant3/1 -> Product2/1
  Mux/1 -> Fr_mp/1
  Constant2/1 -> Mux/1
  Constant4/1 -> Mux/3
  Compare To Zero2/1 -> Product2/2
  Sum2/1 -> Product1/1
  Gain1/1 -> Sum2/2
  Constant1/1 -> Sum2/1
  Sum1/1 -> Product/1
  theta_dot_rp/1 -> Gain1/1, Compare To Zero1/1, Compare To Zero2/1, Compare To Zero/1, Gain/1
  Gain/1 -> Sum1/2
  Constant/1 -> Sum1/1
  Compare To Zero1/1 -> Product1/2
  Compare To Zero/1 -> Product/2

== system constraints_comparison_A_4D_v2_Fc_connected/Subsystem14/Subsystem8 ==
  In1 : Inport
  Demux : Demux  Outputs=7
  Integrator{70..76} (7 alike) : Integrator
  Mux : Mux  Inputs=7
  Out1 : Outport
  wires:
  Mux/1 -> Out1/1
  In1/1 -> Demux/1
  Demux/6 -> Integrator75/1
  Demux/5 -> Integrator74/1
  Demux/4 -> Integrator73/1
  Demux/3 -> Integrator72/1
  Demux/2 -> Integrator71/1
  Demux/7 -> Integrator76/1
  Demux/1 -> Integrator70/1
  Integrator76/1 -> Mux/7
  Integrator75/1 -> Mux/6
  Integrator74/1 -> Mux/5
  Integrator73/1 -> Mux/4
  Integrator72/1 -> Mux/3
  Integrator71/1 -> Mux/2
  Integrator70/1 -> Mux/1

== system constraints_comparison_A_4D_v2_Fc_connected/Subsystem14/Subsystem9 ==
  In1 : Inport
  Angle Conversion : aerolibconvert2/Angle Conversion  IU=deg  OU=rad
  Demux : Demux  Outputs=7
  Demux1 : Demux
  Display : Display
  Integrator70 : Integrator  InitialCondition=-0.672
  Integrator71 : Integrator
  Integrator72 : Integrator
  Integrator73 : Integrator  InitialConditionSource=external  InitialCondition=1
  Integrator74 : Integrator  InitialConditionSource=external
  Integrator75 : Integrator  InitialConditionSource=external
  Integrator76 : Integrator  InitialConditionSource=external
  Mux : Mux  Inputs=7
  Mux2 : Mux  Inputs=3
  Phi : Constant  Value=0
  Psi : Constant  Value=0
  Rotation Angles to Quaternions : sharedtransform/Rotation Angles to Quaternions  rotationOrder=ZYX
      settings: SourceProductName=Aerospace Blockset  SourceProductBaseCode=AE
  Theta : Constant  Value=0
  Out1 : Outport
  wires:
  Angle Conversion/1 -> Rotation Angles to Quaternions/1
  Demux1/3 -> Integrator75/2
  Demux1/2 -> Integrator74/2
  Demux1/1 -> Integrator73/2
  Demux1/4 -> Integrator76/2
  Rotation Angles to Quaternions/1 -> Display/1, Demux1/1
  Mux2/1 -> Angle Conversion/1
  Phi/1 -> Mux2/1
  Psi/1 -> Mux2/3
  Theta/1 -> Mux2/2
  Integrator70/1 -> Mux/1
  Integrator71/1 -> Mux/2
  Integrator72/1 -> Mux/3
  Integrator73/1 -> Mux/4
  Integrator74/1 -> Mux/5
  Integrator75/1 -> Mux/6
  Integrator76/1 -> Mux/7
  Demux/1 -> Integrator70/1
  Demux/7 -> Integrator76/1
  Demux/2 -> Integrator71/1
  Demux/3 -> Integrator72/1
  Demux/4 -> Integrator73/1
  Demux/5 -> Integrator74/1
  Demux/6 -> Integrator75/1
  In1/1 -> Demux/1
  Mux/1 -> Out1/1

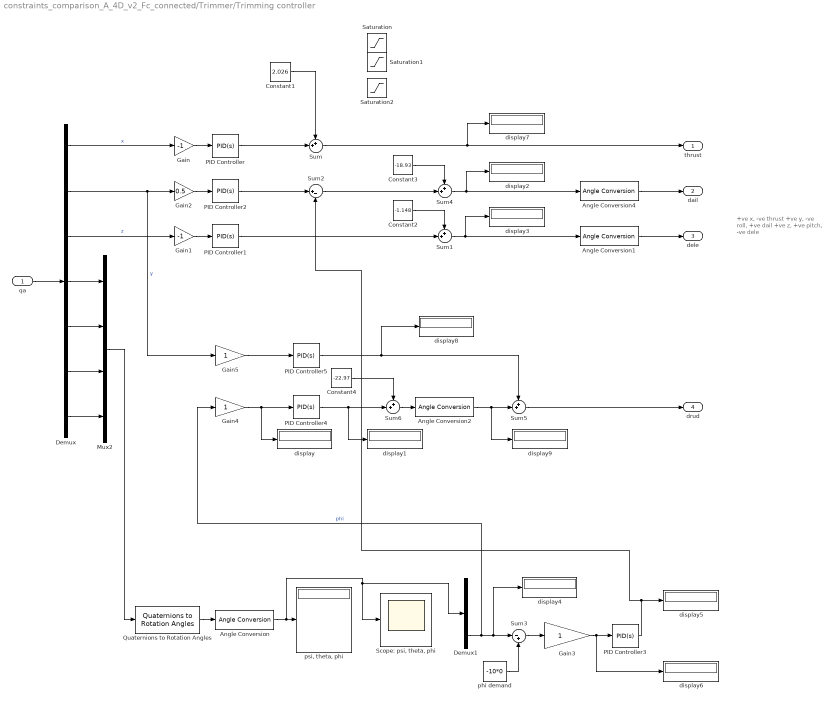
== system constraints_comparison_A_4D_v2_Fc_connected/Trimmer/Trimming controller ==
  note: +ve x, -ve thrust
      |
      | +ve y, -ve roll, +ve dail
      |
      | +ve z, +ve pitch, -ve dele
  qa : Inport
  Angle Conversion : aerolibconvert2/Angle Conversion  IU=rad  OU=deg
  Angle Conversion1 : aerolibconvert2/Angle Conversion  IU=deg  OU=rad
  Angle Conversion2 : aerolibconvert2/Angle Conversion  IU=deg  OU=rad
  Angle Conversion4 : aerolibconvert2/Angle Conversion  IU=deg  OU=rad
  Constant1 : Constant  Value=2.026
  Constant2 : Constant  Value=-1.148
  Constant3 : Constant  Value=-18.93
  Constant4 : Constant  Value=-22.97
  Demux : Demux  Outputs=7
  Demux1 : Demux  Outputs=3
  Gain : Gain  Gain=-1
  Gain1 : Gain  Gain=-1
  Gain2 : Gain  Gain=0.5
  Gain3 : Gain
  Gain4 : Gain
  Gain5 : Gain
  Mux2 : Mux
  PID Controller : simulink/Continuous/PID Controller  Controller=PID  TimeDomain=Continuous-time  SampleTime=-1  IntegratorMethod=Forward Euler  FilterMethod=Forward Euler  Form=Parallel  UseFilter=on  ControllerParametersSource=internal  P=2  I=0.5  D=1  N=100  InitialConditionSource=internal  InitialConditionForIntegrator=0  InitialConditionForFilter=0  ExternalReset=none  LimitOutput=off  UpperSaturationLimit=inf  LowerSaturationLimit=-inf  LinearizeAsGain=on  AntiWindupMode=none  Kb=1  TrackingMode=off  Kt=1  PParamMin=[]  PParamMax=[]  IParamMin=[]  IParamMax=[]  DParamMin=[]  DParamMax=[]  NParamMin=[]  NParamMax=[]  KbParamMin=[]  KbParamMax=[]  KtParamMin=[]  KtParamMax=[]  POutMin=[]  POutMax=[]  IOutMin=[]  IOutMax=[]  DOutMin=[]  DOutMax=[]  NOutMin=[]  NOutMax=[]  KbOutMin=[]  KbOutMax=[]  KtOutMin=[]  KtOutMax=[]  IntegratorOutMin=[]  IntegratorOutMax=[]  FilterOutMin=[]  FilterOutMax=[]  SumOutMin=[]  SumOutMax=[]  SumI1OutMin=[]  SumI1OutMax=[]  SumI2OutMin=[]  SumI2OutMax=[]  SumI3OutMin=[]  SumI3OutMax=[]  SumDOutMin=[]  SumDOutMax=[]  SaturationOutMin=[]  SaturationOutMax=[]  IntegratorContinuousStateAttributes=''  IntegratorStateMustResolveToSignalObject=off  IntegratorRTWStateStorageClass=Auto  FilterContinuousStateAttributes=''  FilterStateMustResolveToSignalObject=off  FilterRTWStateStorageClass=Auto  DifferentiatorICPrevScaledInput=0  DifferentiatorOutMin=[]  DifferentiatorOutMax=[]  InitialConditionSetting=State (most efficient)  FilterDiffOutCoefMin=[]  FilterDiffOutCoefMax=[]  SumDenOutMin=[]  SumDenOutMax=[]  SumNumOutMin=[]  SumNumOutMax=[]  ReciprocalOutMin=[]  ReciprocalOutMax=[]  DivideOutMin=[]  DivideOutMax=[]  TunerSelectOption=Transfer Function Based (PID Tuner App)
  PID Controller1 : simulink/Continuous/PID Controller  Controller=PID  TimeDomain=Continuous-time  SampleTime=-1  IntegratorMethod=Forward Euler  FilterMethod=Forward Euler  Form=Parallel  UseFilter=on  ControllerParametersSource=internal  P=2  I=0.5  D=1  N=100  InitialConditionSource=internal  InitialConditionForIntegrator=0  InitialConditionForFilter=0  ExternalReset=none  LimitOutput=off  UpperSaturationLimit=inf  LowerSaturationLimit=-inf  LinearizeAsGain=on  AntiWindupMode=none  Kb=1  TrackingMode=off  Kt=1  PParamMin=[]  PParamMax=[]  IParamMin=[]  IParamMax=[]  DParamMin=[]  DParamMax=[]  NParamMin=[]  NParamMax=[]  KbParamMin=[]  KbParamMax=[]  KtParamMin=[]  KtParamMax=[]  POutMin=[]  POutMax=[]  IOutMin=[]  IOutMax=[]  DOutMin=[]  DOutMax=[]  NOutMin=[]  NOutMax=[]  KbOutMin=[]  KbOutMax=[]  KtOutMin=[]  KtOutMax=[]  IntegratorOutMin=[]  IntegratorOutMax=[]  FilterOutMin=[]  FilterOutMax=[]  SumOutMin=[]  SumOutMax=[]  SumI1OutMin=[]  SumI1OutMax=[]  SumI2OutMin=[]  SumI2OutMax=[]  SumI3OutMin=[]  SumI3OutMax=[]  SumDOutMin=[]  SumDOutMax=[]  SaturationOutMin=[]  SaturationOutMax=[]  IntegratorContinuousStateAttributes=''  IntegratorStateMustResolveToSignalObject=off  IntegratorRTWStateStorageClass=Auto  FilterContinuousStateAttributes=''  FilterStateMustResolveToSignalObject=off  FilterRTWStateStorageClass=Auto  DifferentiatorICPrevScaledInput=0  DifferentiatorOutMin=[]  DifferentiatorOutMax=[]  InitialConditionSetting=State (most efficient)  FilterDiffOutCoefMin=[]  FilterDiffOutCoefMax=[]  SumDenOutMin=[]  SumDenOutMax=[]  SumNumOutMin=[]  SumNumOutMax=[]  ReciprocalOutMin=[]  ReciprocalOutMax=[]  DivideOutMin=[]  DivideOutMax=[]  TunerSelectOption=Transfer Function Based (PID Tuner App)
  PID Controller2 : simulink/Continuous/PID Controller  Controller=PID  TimeDomain=Continuous-time  SampleTime=-1  IntegratorMethod=Forward Euler  FilterMethod=Forward Euler  Form=Parallel  UseFilter=on  ControllerParametersSource=internal  P=0.1  I=0.1  D=0.5  N=100  InitialConditionSource=internal  InitialConditionForIntegrator=0  InitialConditionForFilter=0  ExternalReset=none  LimitOutput=off  UpperSaturationLimit=inf  LowerSaturationLimit=-inf  LinearizeAsGain=on  AntiWindupMode=none  Kb=1  TrackingMode=off  Kt=1  PParamMin=[]  PParamMax=[]  IParamMin=[]  IParamMax=[]  DParamMin=[]  DParamMax=[]  NParamMin=[]  NParamMax=[]  KbParamMin=[]  KbParamMax=[]  KtParamMin=[]  KtParamMax=[]  POutMin=[]  POutMax=[]  IOutMin=[]  IOutMax=[]  DOutMin=[]  DOutMax=[]  NOutMin=[]  NOutMax=[]  KbOutMin=[]  KbOutMax=[]  KtOutMin=[]  KtOutMax=[]  IntegratorOutMin=[]  IntegratorOutMax=[]  FilterOutMin=[]  FilterOutMax=[]  SumOutMin=[]  SumOutMax=[]  SumI1OutMin=[]  SumI1OutMax=[]  SumI2OutMin=[]  SumI2OutMax=[]  SumI3OutMin=[]  SumI3OutMax=[]  SumDOutMin=[]  SumDOutMax=[]  SaturationOutMin=[]  SaturationOutMax=[]  IntegratorContinuousStateAttributes=''  IntegratorStateMustResolveToSignalObject=off  IntegratorRTWStateStorageClass=Auto  FilterContinuousStateAttributes=''  FilterStateMustResolveToSignalObject=off  FilterRTWStateStorageClass=Auto  DifferentiatorICPrevScaledInput=0  DifferentiatorOutMin=[]  DifferentiatorOutMax=[]  InitialConditionSetting=State (most efficient)  FilterDiffOutCoefMin=[]  FilterDiffOutCoefMax=[]  SumDenOutMin=[]  SumDenOutMax=[]  SumNumOutMin=[]  SumNumOutMax=[]  ReciprocalOutMin=[]  ReciprocalOutMax=[]  DivideOutMin=[]  DivideOutMax=[]  TunerSelectOption=Transfer Function Based (PID Tuner App)
  PID Controller3 : simulink/Continuous/PID Controller  Controller=PID  TimeDomain=Continuous-time  SampleTime=-1  IntegratorMethod=Forward Euler  FilterMethod=Forward Euler  Form=Parallel  UseFilter=on  ControllerParametersSource=internal  P=5  I=0.5  D=2  N=100  InitialConditionSource=internal  InitialConditionForIntegrator=0  InitialConditionForFilter=0  ExternalReset=none  LimitOutput=off  UpperSaturationLimit=inf  LowerSaturationLimit=-inf  LinearizeAsGain=on  AntiWindupMode=none  Kb=1  TrackingMode=off  Kt=1  PParamMin=[]  PParamMax=[]  IParamMin=[]  IParamMax=[]  DParamMin=[]  DParamMax=[]  NParamMin=[]  NParamMax=[]  KbParamMin=[]  KbParamMax=[]  KtParamMin=[]  KtParamMax=[]  POutMin=[]  POutMax=[]  IOutMin=[]  IOutMax=[]  DOutMin=[]  DOutMax=[]  NOutMin=[]  NOutMax=[]  KbOutMin=[]  KbOutMax=[]  KtOutMin=[]  KtOutMax=[]  IntegratorOutMin=[]  IntegratorOutMax=[]  FilterOutMin=[]  FilterOutMax=[]  SumOutMin=[]  SumOutMax=[]  SumI1OutMin=[]  SumI1OutMax=[]  SumI2OutMin=[]  SumI2OutMax=[]  SumI3OutMin=[]  SumI3OutMax=[]  SumDOutMin=[]  SumDOutMax=[]  SaturationOutMin=[]  SaturationOutMax=[]  IntegratorContinuousStateAttributes=''  IntegratorStateMustResolveToSignalObject=off  IntegratorRTWStateStorageClass=Auto  FilterContinuousStateAttributes=''  FilterStateMustResolveToSignalObject=off  FilterRTWStateStorageClass=Auto  DifferentiatorICPrevScaledInput=0  DifferentiatorOutMin=[]  DifferentiatorOutMax=[]  InitialConditionSetting=State (most efficient)  FilterDiffOutCoefMin=[]  FilterDiffOutCoefMax=[]  SumDenOutMin=[]  SumDenOutMax=[]  SumNumOutMin=[]  SumNumOutMax=[]  ReciprocalOutMin=[]  ReciprocalOutMax=[]  DivideOutMin=[]  DivideOutMax=[]  TunerSelectOption=Transfer Function Based (PID Tuner App)
  PID Controller4 : simulink/Continuous/PID Controller  Controller=PID  TimeDomain=Continuous-time  SampleTime=-1  IntegratorMethod=Forward Euler  FilterMethod=Forward Euler  Form=Parallel  UseFilter=on  ControllerParametersSource=internal  P=0.1  I=0  D=0  N=100  InitialConditionSource=internal  InitialConditionForIntegrator=0  InitialConditionForFilter=0  ExternalReset=none  LimitOutput=off  UpperSaturationLimit=inf  LowerSaturationLimit=-inf  LinearizeAsGain=on  AntiWindupMode=none  Kb=1  TrackingMode=off  Kt=1  PParamMin=[]  PParamMax=[]  IParamMin=[]  IParamMax=[]  DParamMin=[]  DParamMax=[]  NParamMin=[]  NParamMax=[]  KbParamMin=[]  KbParamMax=[]  KtParamMin=[]  KtParamMax=[]  POutMin=[]  POutMax=[]  IOutMin=[]  IOutMax=[]  DOutMin=[]  DOutMax=[]  NOutMin=[]  NOutMax=[]  KbOutMin=[]  KbOutMax=[]  KtOutMin=[]  KtOutMax=[]  IntegratorOutMin=[]  IntegratorOutMax=[]  FilterOutMin=[]  FilterOutMax=[]  SumOutMin=[]  SumOutMax=[]  SumI1OutMin=[]  SumI1OutMax=[]  SumI2OutMin=[]  SumI2OutMax=[]  SumI3OutMin=[]  SumI3OutMax=[]  SumDOutMin=[]  SumDOutMax=[]  SaturationOutMin=[]  SaturationOutMax=[]  IntegratorContinuousStateAttributes=''  IntegratorStateMustResolveToSignalObject=off  IntegratorRTWStateStorageClass=Auto  FilterContinuousStateAttributes=''  FilterStateMustResolveToSignalObject=off  FilterRTWStateStorageClass=Auto  DifferentiatorICPrevScaledInput=0  DifferentiatorOutMin=[]  DifferentiatorOutMax=[]  InitialConditionSetting=State (most efficient)  FilterDiffOutCoefMin=[]  FilterDiffOutCoefMax=[]  SumDenOutMin=[]  SumDenOutMax=[]  SumNumOutMin=[]  SumNumOutMax=[]  ReciprocalOutMin=[]  ReciprocalOutMax=[]  DivideOutMin=[]  DivideOutMax=[]  TunerSelectOption=Transfer Function Based (PID Tuner App)
  PID Controller5 : simulink/Continuous/PID Controller  Controller=PID  TimeDomain=Continuous-time  SampleTime=-1  IntegratorMethod=Forward Euler  FilterMethod=Forward Euler  Form=Parallel  UseFilter=on  ControllerParametersSource=internal  P=1.0  I=0.3  D=0.3  N=100  InitialConditionSource=internal  InitialConditionForIntegrator=0  InitialConditionForFilter=0  ExternalReset=none  LimitOutput=off  UpperSaturationLimit=inf  LowerSaturationLimit=-inf  LinearizeAsGain=on  AntiWindupMode=none  Kb=1  TrackingMode=off  Kt=1  PParamMin=[]  PParamMax=[]  IParamMin=[]  IParamMax=[]  DParamMin=[]  DParamMax=[]  NParamMin=[]  NParamMax=[]  KbParamMin=[]  KbParamMax=[]  KtParamMin=[]  KtParamMax=[]  POutMin=[]  POutMax=[]  IOutMin=[]  IOutMax=[]  DOutMin=[]  DOutMax=[]  NOutMin=[]  NOutMax=[]  KbOutMin=[]  KbOutMax=[]  KtOutMin=[]  KtOutMax=[]  IntegratorOutMin=[]  IntegratorOutMax=[]  FilterOutMin=[]  FilterOutMax=[]  SumOutMin=[]  SumOutMax=[]  SumI1OutMin=[]  SumI1OutMax=[]  SumI2OutMin=[]  SumI2OutMax=[]  SumI3OutMin=[]  SumI3OutMax=[]  SumDOutMin=[]  SumDOutMax=[]  SaturationOutMin=[]  SaturationOutMax=[]  IntegratorContinuousStateAttributes=''  IntegratorStateMustResolveToSignalObject=off  IntegratorRTWStateStorageClass=Auto  FilterContinuousStateAttributes=''  FilterStateMustResolveToSignalObject=off  FilterRTWStateStorageClass=Auto  DifferentiatorICPrevScaledInput=0  DifferentiatorOutMin=[]  DifferentiatorOutMax=[]  InitialConditionSetting=State (most efficient)  FilterDiffOutCoefMin=[]  FilterDiffOutCoefMax=[]  SumDenOutMin=[]  SumDenOutMax=[]  SumNumOutMin=[]  SumNumOutMax=[]  ReciprocalOutMin=[]  ReciprocalOutMax=[]  DivideOutMin=[]  DivideOutMax=[]  TunerSelectOption=Transfer Function Based (PID Tuner App)
  Quaternions to Rotation Angles : sharedtransform/Quaternions to Rotation Angles  rotationOrder=ZYX
      settings: SourceProductBaseCode=AE
  Saturation : Saturate  UpperLimit=30*pi/180  LowerLimit=-30*pi/180
  Saturation1 : Saturate  UpperLimit=30*pi/180  LowerLimit=-30*pi/180
  Saturation2 : Saturate  UpperLimit=20*pi/180  LowerLimit=-20*pi/180
  "Scope: psi, theta, phi" : Scope
  Sum{,1,4..6} (5 alike) : Sum  Inputs=++|
  Sum2 : Sum  Inputs=|+-
  Sum3 : Sum  Inputs=|-+
  display{,1..9} (10 alike) : Display
  phi demand : Constant  Value=-10*0
  "psi, theta, phi" : Display
  thrust : Outport
  dail : Outport  Port=2
  dele : Outport  Port=3
  drud : Outport  Port=4
  wires:
  qa/1 -> Demux/1
  Demux/4 -> Mux2/1
  Demux/5 -> Mux2/2
  Demux/6 -> Mux2/3
  Demux/7 -> Mux2/4
  Demux/1 -> Gain/1  "x"
  Demux/2 -> Gain5/1, Gain2/1  "y"
  Demux/3 -> Gain1/1  "z"
  Gain/1 -> PID Controller/1
  Gain1/1 -> PID Controller1/1
  Gain2/1 -> PID Controller2/1
  PID Controller1/1 -> Sum1/2
  Sum/1 -> display7/1, thrust/1
  PID Controller/1 -> Sum/2
  Constant1/1 -> Sum/1
  Sum4/1 -> Angle Conversion4/1, display2/1
  Constant2/1 -> Sum1/1
  Sum1/1 -> Angle Conversion1/1, display3/1
  Angle Conversion4/1 -> dail/1
  Angle Conversion1/1 -> dele/1
  Angle Conversion2/1 -> display9/1, Sum5/2
  Mux2/1 -> Quaternions to Rotation Angles/1
  Quaternions to Rotation Angles/1 -> Angle Conversion/1
  Angle Conversion/1 -> Demux1/1, "Scope: psi, theta, phi"/1, "psi, theta, phi"/1
  PID Controller2/1 -> Sum2/1
  Gain3/1 -> display6/1, PID Controller3/1
  Demux1/3 -> Gain4/1, display4/1, Sum3/1  "phi"
  PID Controller3/1 -> Sum2/2, display5/1
  Sum3/1 -> Gain3/1
  phi demand/1 -> Sum3/2
  Gain4/1 -> PID Controller4/1, display/1
  PID Controller4/1 -> Sum6/2, display1/1
  Sum5/1 -> drud/1
  Gain5/1 -> PID Controller5/1
  PID Controller5/1 -> display8/1, Sum5/1
  Sum2/1 -> Sum4/2
  Constant3/1 -> Sum4/1
  Sum6/1 -> Angle Conversion2/1
  Constant4/1 -> Sum6/1

== system constraints_comparison_A_4D_v2_Fc_connected/Control surface input/1) Short period/2-1-1 ==
  Demux : Demux  Tag=STV Demux  Outputs=1
  FromWs : FromWorkspace  Tag=STV FromWs  VariableName=tuvar  SampleTime=0
      SigBuilderData=|
      | common.afterFinalStr = 'Extrapolate'
      | common.sampleTime = 0
      | dataSet.timeRange = [0 100]
      | dataSet.name = 'Group 1'
      | sbobj.Groups.Name = 'Group 1'
      | sbobj.Groups.Signals.Name = 'Signal 1'
      | sbobj.Groups.Signals.XData = [0 2 2 2.5 2.5 2.75 2.75 3 3 100]
      | sbobj.Groups.Signals.YData = [0 0 -1 -1 1 1 -1 -1 0 0]
      | sbobj.Groups.TimeRange = [0 100]
  Signal 1 : Outport  Tag=STV Outport
  wires:
  Demux/1 -> Signal 1/1
  FromWs/1 -> Demux/1

== system constraints_comparison_A_4D_v2_Fc_connected/Control surface input/1) Short period/3-2-1-1 ==
  Demux : Demux  Tag=STV Demux  Outputs=1
  FromWs : FromWorkspace  Tag=STV FromWs  VariableName=tuvar  SampleTime=0
      SigBuilderData=|
      | common.afterFinalStr = 'Extrapolate'
      | common.sampleTime = 0
      | dataSet.timeRange = [0 100]
      | dataSet.name = 'Group 1'
      | sbobj.Groups.Name = 'Group 1'
      | sbobj.Groups.Signals.Name = 'Signal 1'
      | sbobj.Groups.Signals.XData = [0 2 2 2.75 2.75 3.25 3.25 3.51 3.51 3.75 3.75 100]
      | sbobj.Groups.Signals.YData = [0 0 1 1 -1 -1 1 1 -1 -1 0 0]
      | sbobj.Groups.TimeRange = [0 100]
  Signal 1 : Outport  Tag=STV Outport
  wires:
  FromWs/1 -> Demux/1
  Demux/1 -> Signal 1/1
